simulink model "MotionLab"  (R2024a)
settings: Solver=VariableStepAuto  StartTime=0.0  StopTime=20  RelTol=1e-3  AbsTol=1e-3
values from neighbouring files (symbols this model uses):
  AmplitudeHeave = 0    [HMIVars.m]
  AmplitudePitch = 0    [HMIVars.m]
  AmplitudeRoll = 0    [HMIVars.m]
  AmplitudeSurge = 0    [HMIVars.m]
  AmplitudeSway = 0    [HMIVars.m]
  AmplitudeYaw = 0    [HMIVars.m]
  FrequencyHeave = 0    [HMIVars.m]
  FrequencyPitch = 0    [HMIVars.m]
  FrequencyRoll = 0    [HMIVars.m]
  FrequencySurge = 0    [HMIVars.m]
  FrequencySway = 0    [HMIVars.m]
  FrequencyYaw = 0    [HMIVars.m]
  OffsetHeave = 0    [HMIVars.m]
  OffsetPitch = 0    [HMIVars.m]
  OffsetRoll = 0    [HMIVars.m]
  OffsetSurge = 0    [HMIVars.m]
  OffsetSway = 0    [HMIVars.m]
  OffsetYaw = 0    [HMIVars.m]
  PhaseHeave = 0    [HMIVars.m]
  PhasePitch = 0    [HMIVars.m]
  PhaseRoll = 0    [HMIVars.m]
  PhaseSurge = 0    [HMIVars.m]
  PhaseSway = 0    [HMIVars.m]
  PhaseYaw = 0    [HMIVars.m]
undefined symbols (not defined in the file or in its folder): smiData, smiDataBig, smiDataBigTop, smiDataRobot, Var, X, Y, Z
libraries: sm_lib x438, nesl_utility x74
(part 1 of 14)
settings Model: SimulationMode=accelerator  Creator=thoma  LastModifiedBy=danielh
settings SolverCC: AutoScaleAbsTol=off  AlgebraicLoopSolver=TrustRegion  MaxZcPerStep=1
settings DebuggingCC: UnconnectedInputMsg=warning  UnconnectedOutputMsg=warning  UnconnectedLineMsg=warning  SymbolicDimsDataTypeCodeGenerationDiagnostic=none
settings ModelReferenceCC: EnableRefExpFcnMdlSchedulingChecks=on
settings SFSimCC: CustomCodeUndefinedFunction=UseInterfaceOnly
settings RTWCC: GPUComputeCapability=3.5  DLArmComputeVersion=19.05
settings SimscapeCC: SimscapeLogType=all  SimscapeLogSimulationStatistics=on  SimscapeLogDataHistory=10000

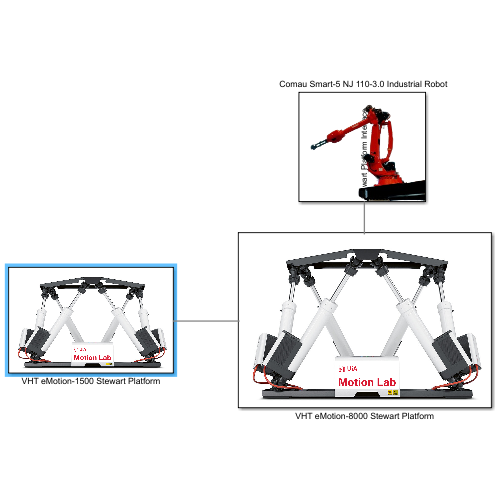
[thumbnail: Simulink's stored preview of the top-level diagram]
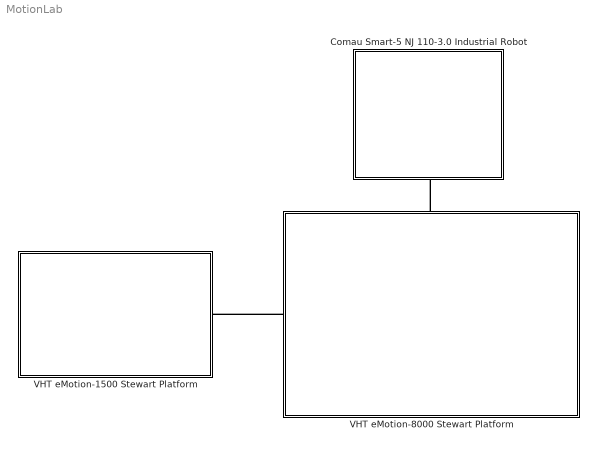
== system MotionLab ==
  " Comau Smart-5 NJ 110-3.0 Industrial Robot" : Subsystem
      settings: PortSchema="{\"entries\":[{\"content\":{\"sides\":[{\"content\":{},\"type\":\"ConnectorPlacement.EquallySpacedRectSide\",\"uuid\":\"640b4a80-a183-4fda-808f-40bbc59803ff\"},{\"content\":{\"side\":\"RIGHT\"},\"type\":\"ConnectorPlacement.EquallySpacedRectSide\",\"uuid\":\"26bc9ede-0f7e-4968-8fcb-4700031f2d04\"},{\"content\":{\"side\":\"TOP\"},\"type\":\"ConnectorPlacement.EquallySpacedRectSide\",\"uuid\":\"f8c1678d-f904-4b2c-ba65-fdabdde128e7\"},{\"content\":{\"connectorIds\":[\"RConn1\"],\"side\":\"BOTTOM\"},\"type\":\"ConnectorPlacement.EquallySpacedRectSide\",\"uuid\":\"31ccf5cf-cde0-4868-907a-e8310ac905dd\"}]},\"type\":\"ConnectorPlacement.EquallySpacedConnector\",\"uuid\":\"53f72707-ebf3-419b-a015-bfc27a2c6f75\"}],\"packageUris\":[\"http://schema.mathworks.com/mf0/Connector/R2020b\"],\"version\":\"1.0\"}"
      mask Display: image('.\Figs\Robot.png');
  VHT eMotion-1500 Stewart Platform : Subsystem
      mask Display: image('.\Figs\StewartPlatform.png');
  VHT eMotion-8000 Stewart Platform : Subsystem
      settings: PortSchema="{\"entries\":[{\"content\":{\"sides\":[{\"content\":{\"connectorIds\":[\"LConn1\"]},\"type\":\"ConnectorPlacement.EquallySpacedRectSide\",\"uuid\":\"db0806e8-caa2-421d-936b-a6f75aa8bfb7\"},{\"content\":{\"side\":\"RIGHT\"},\"type\":\"ConnectorPlacement.EquallySpacedRectSide\",\"uuid\":\"91c2d1eb-1633-461d-b983-e6d74b9ad515\"},{\"content\":{\"connectorIds\":[\"LConn2\"],\"side\":\"TOP\"},\"type\":\"ConnectorPlacement.EquallySpacedRectSide\",\"uuid\":\"8a695272-575a-45c8-aed2-3cc82643c7b5\"}]},\"type\":\"ConnectorPlacement.EquallySpacedConnector\",\"uuid\":\"60269924-cfd7-445e-9c1f-e8fc9453bc0f\"}],\"packageUris\":[\"http://schema.mathworks.com/mf0/Connector/R2020b\"],\"version\":\"1.0\"}"
      mask Display: image('.\Figs\StewartPlatform.png');
  connections:
  VHT eMotion-8000 Stewart Platform/LConn1 -- VHT eMotion-1500 Stewart Platform/RConn1
  VHT eMotion-8000 Stewart Platform/LConn2 -- " Comau Smart-5 NJ 110-3.0 Industrial Robot"/RConn1

== system MotionLab/ Comau Smart-5 NJ 110-3.0 Industrial Robot ==
  PS-Simulink Converter{,1,3..6} (6 alike) : nesl_utility/PS-Simulink Converter  PhysicalDomain=network_engine_domain  SubClassName=ps_output  LeftPortType=input  RightPortType=output  PseudoPeriodic=off  Frequencies=[]  VectorFormat=inherit  Unit=inherit  AffineConversion=off
  Rigid Transform1 : sm_lib/Frames and Transforms/Rigid Transform  RotationMethod=None  FollAlignAxisA=+X  BaseAlignAxisA=+Y  FollAlignAxisB=+Y  BaseAlignAxisB=+Z  RotationStandardAxis=+Z  RotationAngle=0.0  RotationAngleUnits=deg  RotationArbitraryAxis=[0 0 1]  RotationSequenceAxes=FollowerAxes  RotationSequence=XYX  RotationSequenceAngles=[0 0 0]  RotationSequenceAnglesUnits=deg  RotationMatrix=[1 0 0; 0 1 0; 0 0 1]  Quaternion=[1 0 0 0]  TranslationMethod=Cartesian  TranslationCartesianOffset=[-1.1 1.8 0]  TranslationCartesianOffsetUnits=m  TranslationStandardAxis=+Z  TranslationStandardOffset=0  TranslationStandardOffsetUnits=m  TranslationROffset=0  TranslationROffsetUnits=m  TranslationThetaOffset=0  TranslationThetaOffsetUnits=deg  TranslationZOffset=0  TranslationZOffsetUnits=m
  Robot Model : Subsystem
  Terminator{,1..6} (7 alike) : Terminator
  Stewart Platform Interface : PMIOPort  Side=Right
  wires:
  PS-Simulink Converter5/1 -> Terminator5/1  "theta5"
  PS-Simulink Converter4/1 -> Terminator4/1  "theta4"
  PS-Simulink Converter1/1 -> Terminator2/1  "theta2"
  PS-Simulink Converter6/1 -> Terminator6/1  "thet6"
  PS-Simulink Converter/1 -> Terminator/1  "theta1"
  PS-Simulink Converter3/1 -> Terminator3/1  "theta3"
  Robot Model/1(xyz) -> Terminator1/1  "xyz"
  connections:
  Robot Model/RConn4 -- PS-Simulink Converter4/LConn1
  PS-Simulink Converter/LConn1 -- Robot Model/RConn1
  Robot Model/RConn6 -- PS-Simulink Converter6/LConn1
  Robot Model/RConn3 -- PS-Simulink Converter3/LConn1
  Robot Model/RConn5 -- PS-Simulink Converter5/LConn1
  PS-Simulink Converter1/LConn1 -- Robot Model/RConn2
  Rigid Transform1/RConn1 -- Robot Model/LConn1
  Stewart Platform Interface/RConn1 -- Rigid Transform1/LConn1

== system MotionLab/VHT eMotion-1500 Stewart Platform ==
  ExtractAndCombinePosAndVel1 : Subsystem
  Inverse Kinematics1 : Subsystem
  Motion Control System : Subsystem
  Rigid Transform : sm_lib/Frames and Transforms/Rigid Transform  RotationMethod=None  FollAlignAxisA=+X  BaseAlignAxisA=+Y  FollAlignAxisB=+Y  BaseAlignAxisB=+Z  RotationStandardAxis=+Z  RotationAngle=0.0  RotationAngleUnits=deg  RotationArbitraryAxis=[0 0 1]  RotationSequenceAxes=FollowerAxes  RotationSequence=XYX  RotationSequenceAngles=[0 0 0]  RotationSequenceAnglesUnits=deg  RotationMatrix=[1 0 0; 0 1 0; 0 0 1]  Quaternion=[1 0 0 0]  TranslationMethod=Cartesian  TranslationCartesianOffset=[-3 4 0]  TranslationCartesianOffsetUnits=m  TranslationStandardAxis=+Z  TranslationStandardOffset=0  TranslationStandardOffsetUnits=m  TranslationROffset=0  TranslationROffsetUnits=m  TranslationThetaOffset=0  TranslationThetaOffsetUnits=deg  TranslationZOffset=0  TranslationZOffsetUnits=m
  Terminator{,1..6} (7 alike) : Terminator
  UiA Stewart Platform1 : Subsystem
      settings: PortSchema="{\"entries\":[{\"content\":{\"sides\":[{\"content\":{\"connectorIds\":[\"In1\",\"In2\",\"In3\",\"In4\",\"In5\",\"In6\"]},\"type\":\"ConnectorPlacement.EquallySpacedRectSide\",\"uuid\":\"7f0ff7fd-0348-45ad-beb9-8ad2ec3e2887\"},{\"content\":{\"connectorIds\":[\"Out1\",\"Out2\",\"Out3\",\"Out4\",\"Out5\",\"Out6\",\"Out7\",\"Out8\",\"Out9\",\"Out10\"],\"side\":\"RIGHT\"},\"type\":\"ConnectorPlacement.EquallySpacedRectSide\",\"uuid\":\"276042a1-7937-4cae-810e-b80b5f2637b1\"},{\"content\":{\"connectorIds\":[\"LConn1\"],\"side\":\"TOP\"},\"type\":\"ConnectorPlacement.EquallySpacedRectSide\",\"uuid\":\"d74fb182-1c8f-4c06-a6da-c93034697881\"}]},\"type\":\"ConnectorPlacement.EquallySpacedConnector\",\"uuid\":\"3d2973ff-43c5-4cbf-9014-0a5cde3717a6\"}],\"packageUris\":[\"http://schema.mathworks.com/mf0/Connector/R2020b\"],\"version\":\"1.0\"}"
  MBS Config : PMIOPort  Side=Right
  wires:
  UiA Stewart Platform1/1("xCyl1, vCyl1, fCyl1") -> ExtractAndCombinePosAndVel1/1(In1)
  Motion Control System/6(xRefCyl6) -> UiA Stewart Platform1/6(xRefCyl6)
  Motion Control System/5(xRefCyl5) -> UiA Stewart Platform1/5(xRefCyl5)
  Motion Control System/9(ptop) -> Inverse Kinematics1/3(pos)
  Motion Control System/8(w_top) -> Inverse Kinematics1/2(w)
  Motion Control System/4(xRefCyl4) -> UiA Stewart Platform1/4(xRefCyl4)
  UiA Stewart Platform1/6("xCyl6, vCyl6, fCyl6") -> ExtractAndCombinePosAndVel1/6(In6)
  Motion Control System/2(xRefCyl2) -> UiA Stewart Platform1/2(xRefCyl2)
  Motion Control System/3(xRefCyl3) -> UiA Stewart Platform1/3(xRefCyl3)
  UiA Stewart Platform1/7(R) -> Terminator/1
  Motion Control System/7(R_top) -> Inverse Kinematics1/1(Rot)
  UiA Stewart Platform1/3("xCyl3, vCyl3, fCyl3") -> ExtractAndCombinePosAndVel1/3(In3)
  UiA Stewart Platform1/8(w) -> Terminator1/1
  Motion Control System/1(xRefCyl1) -> UiA Stewart Platform1/1(xRefCyl1)
  UiA Stewart Platform1/4("xCyl4, vCyl4, fCyl4") -> ExtractAndCombinePosAndVel1/4(In4)
  UiA Stewart Platform1/10(v) -> Terminator5/1
  Motion Control System/10(v_top) -> Inverse Kinematics1/4(vel)
  UiA Stewart Platform1/9(p) -> Terminator2/1
  UiA Stewart Platform1/2("xCyl2, vCyl2, fCyl2") -> ExtractAndCombinePosAndVel1/2(In2)
  UiA Stewart Platform1/5("xCyl5, vCyl5, fCyl5") -> ExtractAndCombinePosAndVel1/5(In5)
  Inverse Kinematics1/1(y) -> Motion Control System/1(DesiredPos)
  Inverse Kinematics1/2(y1) -> Terminator3/1
  ExtractAndCombinePosAndVel1/2(ActualLegVel) -> Terminator4/1
  ExtractAndCombinePosAndVel1/1(ActualLegPos) -> Terminator6/1
  connections:
  Rigid Transform/RConn1 -- UiA Stewart Platform1/LConn1
  MBS Config/RConn1 -- Rigid Transform/LConn1

== system MotionLab/VHT eMotion-8000 Stewart Platform ==
  ExtractAndCombinePosAndVel : Subsystem
  Inverse Kinematics : Subsystem
  MBS Config : Subsystem
  Motion Control System : Subsystem
  Terminator{,1..6} (7 alike) : Terminator
  UiA Stewart Platform : Subsystem
      settings: PortSchema="{\"entries\":[{\"content\":{\"sides\":[{\"content\":{\"connectorIds\":[\"In1\",\"In2\",\"In3\",\"In4\",\"In5\",\"In6\"]},\"type\":\"ConnectorPlacement.EquallySpacedRectSide\",\"uuid\":\"de8fd662-7a9e-4209-b357-dad0c75e3639\"},{\"content\":{\"connectorIds\":[\"Out1\",\"Out2\",\"Out3\",\"Out4\",\"Out5\",\"Out6\",\"Out7\",\"Out8\",\"Out9\",\"Out10\"],\"side\":\"RIGHT\"},\"type\":\"ConnectorPlacement.EquallySpacedRectSide\",\"uuid\":\"e834d12e-6262-442b-ab59-0eaa631772a0\"},{\"content\":{\"connectorIds\":[\"LConn1\",\"LConn2\"],\"side\":\"TOP\"},\"type\":\"ConnectorPlacement.EquallySpacedRectSide\",\"uuid\":\"a8020181-8251-4e51-94b7-b1fc3bb6a903\"}]},\"type\":\"ConnectorPlacement.EquallySpacedConnector\",\"uuid\":\"4c8cdd83-1355-404f-82e4-691ae5a3080a\"}],\"packageUris\":[\"http://schema.mathworks.com/mf0/Connector/R2020b\"],\"version\":\"1.0\"}"
  eMotion-1500 Interface : PMIOPort  Side=Left
  Robot Interface : PMIOPort  Port=2  Side=Left
  wires:
  Motion Control System/3(xRefCyl3) -> UiA Stewart Platform/3(xRefCyl3)
  Motion Control System/9(ptop) -> Inverse Kinematics/3(posBig)
  Motion Control System/10(v_top) -> Inverse Kinematics/4(velBig)
  Motion Control System/6(xRefCyl6) -> UiA Stewart Platform/6(xRefCyl6)
  Motion Control System/5(xRefCyl5) -> UiA Stewart Platform/5(xRefCyl5)
  UiA Stewart Platform/9(pBig) -> Terminator4/1
  UiA Stewart Platform/4("xCyl4, vCyl4, fCyl1") -> ExtractAndCombinePosAndVel/4(In4)
  UiA Stewart Platform/7(RBig) -> Terminator/1
  Motion Control System/2(xRefCyl2) -> UiA Stewart Platform/2(xRefCyl2)
  UiA Stewart Platform/10(vBig) -> Terminator5/1
  UiA Stewart Platform/8(wBig) -> Terminator3/1
  Motion Control System/7(R_top) -> Inverse Kinematics/1(RotBig)
  UiA Stewart Platform/6("xCyl6, vCyl6, fCyl1") -> ExtractAndCombinePosAndVel/6(In6)
  Motion Control System/4(xRefCyl4) -> UiA Stewart Platform/4(xRefCyl4)
  Motion Control System/8(w_top) -> Inverse Kinematics/2(wBig)
  UiA Stewart Platform/1("xCyl1, vCyl1, fCyl2") -> ExtractAndCombinePosAndVel/1(In1)
  UiA Stewart Platform/2("xCyl2, vCyl2, fCyl1") -> ExtractAndCombinePosAndVel/2(In2)
  UiA Stewart Platform/3("xCyl3, vCyl3, fCyl1") -> ExtractAndCombinePosAndVel/3(In3)
  Motion Control System/1(xRefCyl1) -> UiA Stewart Platform/1(xRefCyl1)
  Inverse Kinematics/1(y) -> Motion Control System/1(DesiredPos)
  UiA Stewart Platform/5("xCyl5, vCyl5, fCyl1") -> ExtractAndCombinePosAndVel/5(In5)
  Inverse Kinematics/2(y1) -> Terminator1/1
  ExtractAndCombinePosAndVel/2(ActualLegVel) -> Terminator2/1
  ExtractAndCombinePosAndVel/1(ActualLegPos) -> Terminator6/1
  connections:
  Robot Interface/RConn1 -- UiA Stewart Platform/LConn1
  eMotion-1500 Interface/RConn1 -- MBS Config/RConn1 -- UiA Stewart Platform/LConn2
